simulink model "SPMS"  (R2019a)
settings: Solver=FixedStepAuto  StartTime=0.0  StopTime=inf  RelTol=1e-3  EnableMultiTasking=on
libraries: arduinolib x5, simulink x2, LCDlib x1
settings Model: SimulationMode=external  ExtModeTrigDuration=2  Creator=hp  LastModifiedBy=rishi
settings OptimizationCC: EnhancedBackFolding=on  PassReuseOutputArgsAs=Individual arguments  MaxStackSize=64  OptimizeBlockOrder=speed  DifferentSizesBufferReuse=on  OptimizationCustomize=off
settings DebuggingCC: ParameterTunabilityLossMsg=error
settings HardwareCC: ProdBitPerInt=16  ProdBitPerPointer=16  ProdBitPerSizeT=16  ProdBitPerPtrDiffT=16  ProdLargestAtomicFloat=None  ProdWordSize=8  ProdHWDeviceType=Atmel->AVR
settings SFSimCC: MATLABDynamicMemAlloc=off
settings RTWCC: SystemTargetFile=ert.tlc  HardwareBoard=Arduino Uno  TLCOptions=-aInlineSetEventsForThisBaseRateFcn=TLC_FALSE -aSuppressMultiTaskScheduler=TLC_FALSE -aRateBasedStepFcn=1  TemplateMakefile=ert_default_tmf  GenerateReport=on  Toolchain=Arduino AVR  BuildConfiguration=Faster Runs  IncludeHyperlinkInReport=on  LaunchReport=on  GenerateTraceInfo=on  GenerateTraceReport=on  GenerateTraceReportSl=on  GenerateTraceReportSf=on  GenerateTraceReportEml=on
settings CodeAppCC: ForceParamTrailComments=on  IgnoreCustomStorageClasses=off  OperatorAnnotations=on  SimulinkDataObjDesc=on  SFDataObjDesc=on  InsertBlockDesc=on
settings ERTTargetCC: SupportContinuousTime=on  SupportVariableSizeSignals=on  ExtMode=on  ExtModeStaticAllocSize=250  ExtModeMexArgs='127.0.0.1' 0 17725

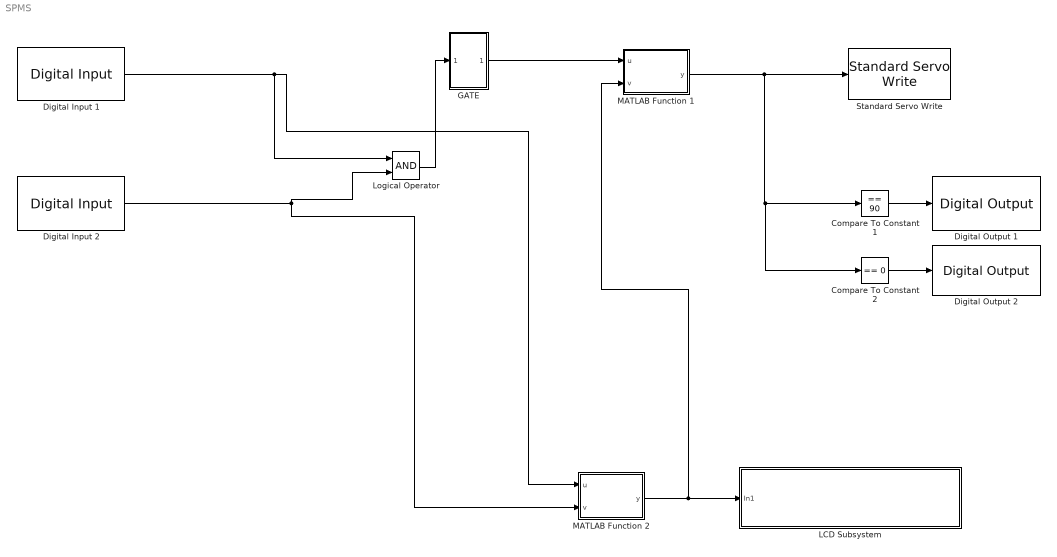
== system SPMS ==
  Compare To Constant 1 : simulink/Logic and Bit Operations/Compare To Constant  relop===  const=90  OutDataTypeStr=boolean
  Compare To Constant 2 : simulink/Logic and Bit Operations/Compare To Constant  relop===  const=0  OutDataTypeStr=boolean
  Digital Input 1 : arduinolib/Digital Input  pinNumber=12  sampleTime=1  blockPlatform=arduino
      settings: SourceProductName=Simulink Support Package for Arduino Hardware
  Digital Input 2 : arduinolib/Digital Input  pinNumber=13  sampleTime=1  blockPlatform=arduino
      settings: SourceProductName=Simulink Support Package for Arduino Hardware
  Digital Output 1 : arduinolib/Digital Output  pinNumber=3  blockPlatform=arduino
  Digital Output 2 : arduinolib/Digital Output  pinNumber=2  blockPlatform=arduino
  GATE : Subsystem
  LCD Subsystem : Subsystem
  Logical Operator : Logic  AllPortsSameDT=off  OutDataTypeStr=boolean
  MATLAB Function 1 : MATLAB Function  TreatAsAtomicUnit=on
  MATLAB Function 2 : MATLAB Function  TreatAsAtomicUnit=on
  Standard Servo Write : arduinolib/Standard Servo Write  pinNumber=9  ServoIndex=0  blockPlatform=ARDUINO
      settings: SourceProductName=Simulink Support Package for Arduino Hardware
  wires:
  Logical Operator/1 -> GATE/1(In1)
  Digital Input 2/1 -> MATLAB Function 2/2(v), Logical Operator/2
  Digital Input 1/1 -> MATLAB Function 2/1(u), Logical Operator/1
  Compare To Constant 1/1 -> Digital Output 1/1
  Compare To Constant 2/1 -> Digital Output 2/1
  MATLAB Function 2/1(y) -> LCD Subsystem/1(In1), MATLAB Function 1/2(v)
  GATE/1(Out1) -> MATLAB Function 1/1(u)
  MATLAB Function 1/1(y) -> Compare To Constant 2/1, Compare To Constant 1/1, Standard Servo Write/1

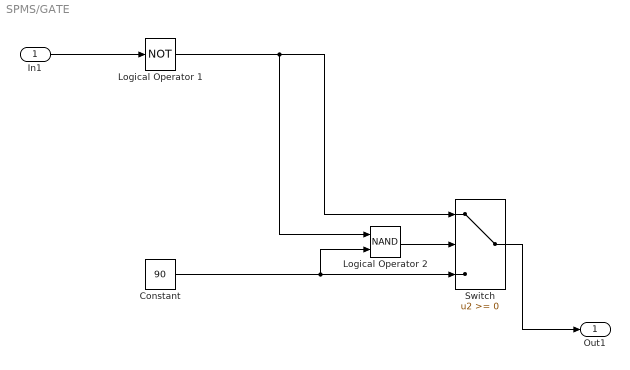
== system SPMS/GATE ==
  In1 : Inport
  Constant : Constant  Value=90  VectorParams1D=off
  Logical Operator 1 : Logic  Operator=NOT  Inputs=1  AllPortsSameDT=off  OutDataTypeStr=boolean
  Logical Operator 2 : Logic  Operator=NAND  AllPortsSameDT=off  OutDataTypeStr=boolean
  Switch : Switch
  Out1 : Outport
  wires:
  Switch/1 -> Out1/1
  Constant/1 -> Logical Operator 2/2, Switch/3
  Logical Operator 2/1 -> Switch/2
  Logical Operator 1/1 -> Logical Operator 2/1, Switch/1
  In1/1 -> Logical Operator 1/1

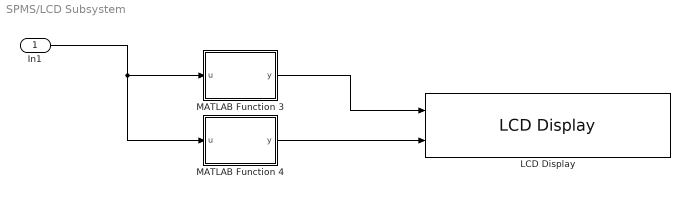
== system SPMS/LCD Subsystem ==
  In1 : Inport
  LCD Display : LCDlib/LCD Display  pins=[11,10,7,6,5,4]
      settings: SourceProductName=LCD Library
  MATLAB Function 3 : MATLAB Function  TreatAsAtomicUnit=on
  MATLAB Function 4 : MATLAB Function  TreatAsAtomicUnit=on
  wires:
  MATLAB Function 4/1(y) -> LCD Display/2
  MATLAB Function 3/1(y) -> LCD Display/1
  In1/1 -> MATLAB Function 4/1(u), MATLAB Function 3/1(u)

== matlab function SPMS/LCD Subsystem/MATLAB Function 4 ==
  data: u input; y output
function y = fcn(u)
if u<0
    u = 0;
elseif u>13
    u = 13;
end
switch u
    case 13
        y=[78 111 46 32 111 102 32 115 112 111 116 115 58 32 49 51];
    case 12
        y=[78 111 46 32 111 102 32 115 112 111 116 115 58 32 49 50];
    case 11
        y=[78 111 46 32 111 102 32 115 112 111 116 115 58 32 49 49];
    case 10
        y=[78 111 46 32 111 102 32 115 112 111 116 115 58 32 49 48];
    case 9
        y=[78 111 46 32 111 102 32 115 112 111 116 115 58 32 48 57];
    case 8
        y=[78 111 46 32 111 102 32 115 112 111 116 115 58 32 48 56];
    case 7
        y=[78 111 46 32 111 102 32 115 112 111 116 115 58 32 48 55];
    case 6
        y=[78 111 46 32 111 102 32 115 112 111 116 115 58 32 48 54];
    case 5
        y=[78 111 46 32 111 102 32 115 112 111 116 115 58 32 48 53];
    case 4
        y=[78 111 46 32 111 102 32 115 112 111 116 115 58 32 48 52];
    case 3
        y=[78 111 46 32 111 102 32 115 112 111 116 115 58 32 48 51];
    case 2
       y=[78 111 46 32 111 102 32 115 112 111 116 115 58 32 48 50];
    case 1
        y=[78 111 46 32 111 102 32 115 112 111 116 115 58 32 48 49];
    otherwise 
        y=[78 111 46 32 111 102 32 115 112 111 116 115 58 32 48 48];
end

== matlab function SPMS/LCD Subsystem/MATLAB Function 3 ==
  data: u input; y output
function y = fcn(u)
if u>0
    y=[87 101 108 99 111 109 101 32 32 32 32 32 32 32 32];
else 
    y=[80 108 122 46 32 99 111 109 101 32 108 97 116 101 114];
end

== matlab function SPMS/MATLAB Function 2 ==
  data: u input; y output; v input
function y = fcn(u,v)
persistent n;
total = 13;
if isempty(n)
    n = 0;
end
if u==0
    n = n+1;
elseif v==0
    n = n-1;
end
y = total - n;
if y>13
    n=0;
elseif y<0
    n=13;
end

== matlab function SPMS/MATLAB Function 1 ==
  data: u input; y output; v input
function y = fcn(u,v)
if v<=13 && v>=0
    y = u;
else
    y = 0;
end
